simulink model "ex2"  (Simulink 6.0)
settings: Solver=ode45  StartTime=0.0  StopTime=10.0  RelTol=1e-3
values from neighbouring files (symbols this model uses):
  hn_hpf = fir1(N-1, Wcn, 'high')    [ex2_simu.m]
  hn_lpf = fir1(N-1, Wcn)    [ex2_simu.m]
settings Model: LastModifiedBy=student

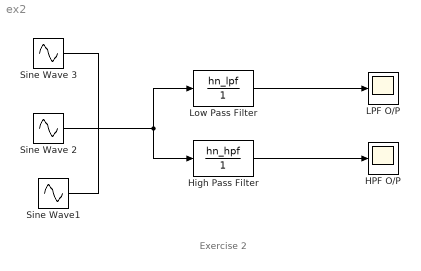
== system ex2 ==
  note: Exercise 2
  HPF O/P : Scope
  High Pass Filter : DiscreteFilter  Numerator=hn_hpf  Denominator=1
  LPF O/P : Scope
  Low Pass Filter : DiscreteFilter  Numerator=hn_lpf  Denominator=1  SampleTime=0.0001
  Sine Wave 2 : Sin  Frequency=pi * 3600  SampleTime=0.0001
  Sine Wave 3 : Sin  Frequency=pi * 3600  SampleTime=0.0001
  Sine Wave1 : Sin  Amplitude=2  Frequency=pi * 5000  SampleTime=0.0001
  wires:
  Sine Wave 2/1 -> Low Pass Filter/1, High Pass Filter/1
  Sine Wave 3/1 -> ?
  Sine Wave1/1 -> ?
  Low Pass Filter/1 -> LPF O/P/1
  High Pass Filter/1 -> HPF O/P/1
